simulink model "c10mfode4"  (Simulink 7.7)
settings: Solver=ode15s  StartTime=0.0  StopTime=10  RelTol=1e-6
PreLoadFcn:
  | ww=[1e-3,1e3];
settings Model: Creator=Professor Dingyu Xue  LastModifiedBy=Professor Dingyu Xue
settings DataIOCC: LimitDataPoints=off  SignalLoggingName=sigsOut
settings DebuggingCC: SaveWithParameterizedLinksMsg=none  SignalResolutionControl=TryResolveAllWithWarning  SolverPrmCheckMsg=none  MultiTaskDSMMsg=warning  MultiTaskCondExecSysMsg=none  StrictBusMsg=None
settings HardwareCC: TargetUnknown=on
settings RTWCC: IncludeERTFirstTime=on

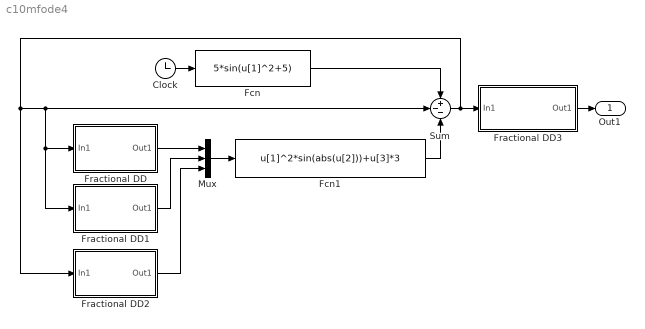
== system c10mfode4 ==
  Clock : Clock
      settings: Decimation=10
  Fcn : Fcn  Expr=5*sin(u[1]^2+5)
  Fcn1 : Fcn  Expr=u[1]^2*sin(abs(u[2]))+u[3]*3
  Fractional DD : Subsystem  mask{gam=0.6, ww=ww, n=4}
      mask prompts: gam "Derivative order gamma"; ww "Frequency range [wb,wh]"; n "Apprixmation order"
      mask init:
      | wb=ww(1); wh=ww(2); G=ousta_fod(gam,n,wb,wh);
      | num=G.num{1}; den=G.den{1}; T=1/wh; str='Fractional\n';
      | if isnumeric(gam)
      | 	if gam>0, str=[str, 'Der  s^' num2str(gam) ];
      | 	else, str=[str, 'Int  s^{' num2str(gam) '}']; end
      | else, str=[str, 'Der  s^gam']; end
      mask Display: disp(str)
  Fractional DD1 : Subsystem  mask{gam=0.8, ww=ww, n=4}
      mask prompts: gam "Derivative order gamma"; ww "Frequency range [wb,wh]"; n "Apprixmation order"
      mask init: same as c10mfode4/Fractional DD
      mask Display: disp(str)
  Fractional DD2 : Subsystem  mask{gam=0.2, ww=ww, n=4}
      mask prompts: gam "Derivative order gamma"; ww "Frequency range [wb,wh]"; n "Apprixmation order"
      mask init: same as c10mfode4/Fractional DD
      mask Display: disp(str)
  Fractional DD3 : Subsystem  mask{gam=-0.2, ww=ww, n=4}
      mask prompts: gam "Derivative order gamma"; ww "Frequency range [wb,wh]"; n "Apprixmation order"
      mask init: same as c10mfode4/Fractional DD
      mask Display: disp(str)
  Mux : Mux  Inputs=3
  Sum : Sum  Inputs=+--  SaturateOnIntegerOverflow=on
  Out1 : Outport
  wires:
  Fractional DD1/1(Out1) -> Mux/2
  Fractional DD2/1(Out1) -> Mux/3
  Sum/1 -> Sum/2, Fractional DD/1(In1), Fractional DD1/1(In1), Fractional DD2/1(In1), Fractional DD3/1(In1)
  Clock/1 -> Fcn/1
  Fcn/1 -> Sum/1
  Fractional DD3/1(Out1) -> Out1/1
  Fractional DD/1(Out1) -> Mux/1
  Mux/1 -> Fcn1/1
  Fcn1/1 -> Sum/3

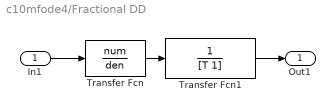
== system c10mfode4/Fractional DD ==
  In1 : Inport
  Transfer Fcn : TransferFcn  Numerator=num  Denominator=den
  Transfer Fcn1 : TransferFcn  Numerator=1  Denominator=[T 1]
  Out1 : Outport
  wires:
  In1/1 -> Transfer Fcn/1
  Transfer Fcn/1 -> Transfer Fcn1/1
  Transfer Fcn1/1 -> Out1/1

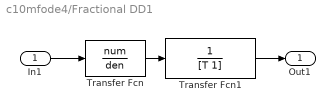
== system c10mfode4/Fractional DD1 ==
  In1 : Inport
  Transfer Fcn : TransferFcn  Numerator=num  Denominator=den
  Transfer Fcn1 : TransferFcn  Numerator=1  Denominator=[T 1]
  Out1 : Outport
  wires:
  Transfer Fcn1/1 -> Out1/1
  Transfer Fcn/1 -> Transfer Fcn1/1
  In1/1 -> Transfer Fcn/1

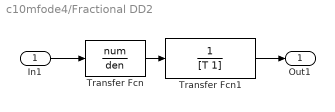
== system c10mfode4/Fractional DD2 ==
  In1 : Inport
  Transfer Fcn : TransferFcn  Numerator=num  Denominator=den
  Transfer Fcn1 : TransferFcn  Numerator=1  Denominator=[T 1]
  Out1 : Outport
  wires:
  In1/1 -> Transfer Fcn/1
  Transfer Fcn/1 -> Transfer Fcn1/1
  Transfer Fcn1/1 -> Out1/1

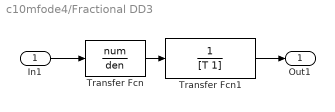
== system c10mfode4/Fractional DD3 ==
  In1 : Inport
  Transfer Fcn : TransferFcn  Numerator=num  Denominator=den
  Transfer Fcn1 : TransferFcn  Numerator=1  Denominator=[T 1]
  Out1 : Outport
  wires:
  In1/1 -> Transfer Fcn/1
  Transfer Fcn/1 -> Transfer Fcn1/1
  Transfer Fcn1/1 -> Out1/1
